simulink model "Single_phase_full_wave_full_controlled_rectifier"  (R2022b)
settings: Solver=VariableStepAuto  StartTime=0.0  StopTime=0.5  RelTol=1e-3
libraries: spsThyristorLib x4, spsVoltageMeasurementLib x2, spsACVoltageSourceLib x1, spsDiodeLib x1, spsSeriesRLCBranchLib x1, sps_lib x1
settings Model: Creator=Biplov Jha  LastModifiedBy=Biplov Jha

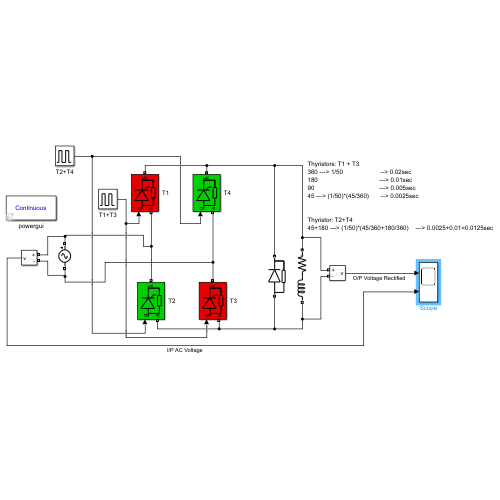
[thumbnail: Simulink's stored preview of the top-level diagram]
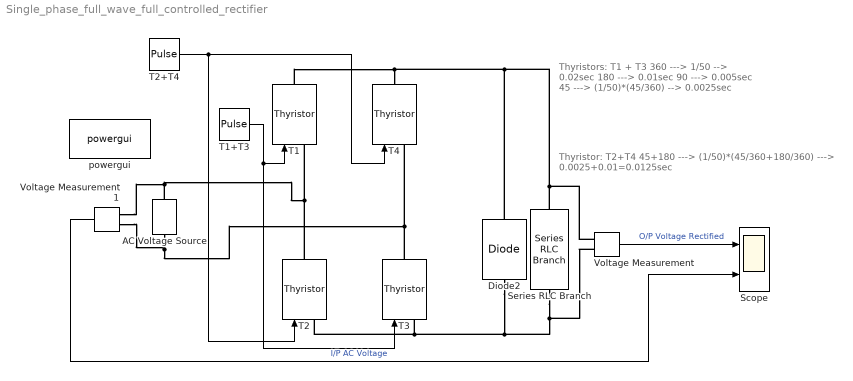
== system Single_phase_full_wave_full_controlled_rectifier ==
  note: Thyristor: T2+T4
      | 45+180 ---> (1/50)*(45/360+180/360)    ---> 0.0025+0.01=0.0125sec
  note: Thyristors: T1 + T3
      | 360 ---> 1/50                      --> 0.02sec
      | 180                                    ---> 0.01sec
      | 90                                      ---> 0.005sec
      | 45 ---> (1/50)*(45/360)       --> 0.0025sec
  AC Voltage Source : spsACVoltageSourceLib/AC Voltage Source  Amplitude=325  Phase=0  Frequency=50  SampleTime=0  Measurements=None  BusType=swing  Pref=10e3  Qref=0  Qmin=-inf  Qmax=+inf
  Diode2 : spsDiodeLib/Diode  Ron=0.001  Lon=0  Vf=0.8  IC=0  UseSnubber=0  Rs=500  Cs=250e-9  Measurements=off
  Scope : Scope  NumInputPorts=2
  Series RLC Branch : spsSeriesRLCBranchLib/Series RLC Branch  LConnTagsString=__new0  RConnTagsString=__new0  BranchType=RL  Resistance=0.5  Inductance=650e-3  SetiL0=off  InitialCurrent=0  Capacitance=1e-6  Setx0=off  InitialVoltage=0  Measurements=None
  T{1..4} (4 alike) : spsThyristorLib/Thyristor  Ron=0.001  Lon=0  Vf=0.8  IC=0  Rs=500  Cs=250e-9  Measurements=off
  T1+T3 : DiscretePulseGenerator  PulseType=Time based  Period=1/50  PulseWidth=5  PhaseDelay=(1/50)*(90/360)
  T2+T4 : DiscretePulseGenerator  PulseType=Time based  Period=1/50  PulseWidth=5  PhaseDelay=(1/50)*(45/360+180/360)
  Voltage Measurement : spsVoltageMeasurementLib/Voltage Measurement  PhasorSimulation=off  OutputType=Complex  PSBequivalent=0
  Voltage Measurement1 : spsVoltageMeasurementLib/Voltage Measurement  PhasorSimulation=off  OutputType=Complex  PSBequivalent=0
  powergui : sps_lib/powergui  Priority=1  SimulationMode=Continuous  SampleTime=50e-6  frequency=60  Iterations=50  frequencyindice=50  Pbase=100e6  ErrMax=1e-4  UnitsV=kV  UnitsW=MW  buscounter=0  FunctionMessages=off  echomessages=off  EnableUseOfTLC=off  CurrentSourceSwitches=off  DisableSnubberDevices=off  DisableRonSwitches=off  DisableVfSwitches=off  DisplayEquations=off  AutomaticDiscreteSolvers=off  SolverType=Tustin/Backward Euler (TBE)  Interpol=off  ExternalGateDelay=off  methode=off  Ts=100  x0status=blocks  SPID=on  SwTol=0  HookPort=off  NonlinearTolerance=1e-4  nMaxIteration=100  ContinueOnMaxIteration=off  RestoreLinks=warning  ResistiveCurrentMeasurement=off  Frange=[0:2:500]  Ylog=off  Xlog=on  ShowGrid=off  save=off  variable=ZData  structure=0  ZoomFFT=off  StartTime=0.0  cycles=1  DisplayStyle=1  fundamental=60  FreqAxis=off  MaxFrequency=1000  frequencyindicesteady=1  RmsSteady=1  display=off
  wires:
  Voltage Measurement/1 -> Scope/1  "O/P Voltage Rectified"
  Voltage Measurement1/1 -> Scope/2  "I/P AC Voltage"
  T1+T3/1 -> T3/1, T1/1
  T2+T4/1 -> T4/1, T2/1
  connections:
  T1/LConn1 -- T2/RConn1 -- Voltage Measurement1/LConn1 -- AC Voltage Source/RConn1
  T4/LConn1 -- T3/RConn1 -- Voltage Measurement1/LConn2 -- AC Voltage Source/LConn1
  T1/RConn1 -- Voltage Measurement/LConn1 -- Series RLC Branch/LConn1 -- Diode2/RConn1 -- T4/RConn1
  Series RLC Branch/RConn1 -- Voltage Measurement/LConn2 -- Diode2/LConn1 -- T2/LConn1 -- T3/LConn1
